simulink model "mainModel"  (R2018a)
settings: Solver=ode4  StartTime=0.0  StopTime=tsim  FixedStep=dt  RelTol=1e-3
values from neighbouring files (symbols this model uses):
  bh = 1.72    [loadParameters.m]
  Bm = 0.101    [loadParameters.m]
  Bs = 0.0602    [loadParameters.m]
  Im = 0.00136    [loadParameters.m]
  Is = 0.00129    [loadParameters.m]
  Kd = 0.1    [main.m]
  kh = 155    [loadParameters.m]
  Kp = 1.0    (= 1)    [main.m]
  L = 0.075    [loadParameters.m]
  mh = 0.1    [loadParameters.m]
  OPTION = 2    [main.m]
  wph = 87.3    [loadParameters.m]
  wzh = 98.7    [loadParameters.m]
  zph = 0.49    [loadParameters.m]
libraries: simulink_extras x1
settings Model: Creator=s118759  LastModifiedBy=s118759
settings DebuggingCC: AlgebraicLoopMsg=none

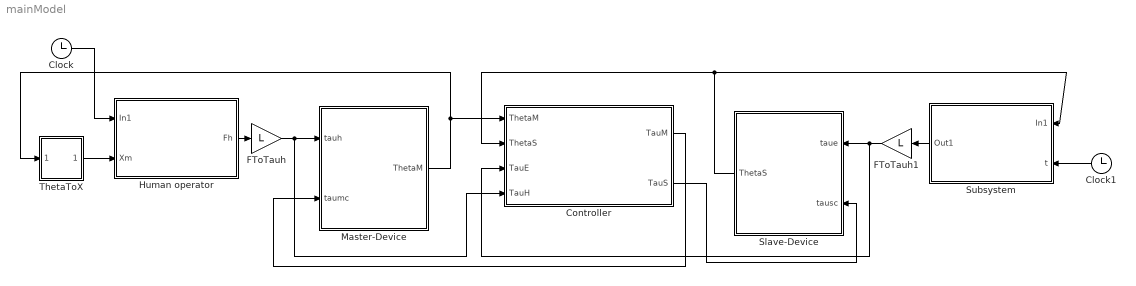
== system mainModel ==
  Clock : Clock
  Clock1 : Clock
  "Controller " : Subsystem
  FToTauh : Gain  Gain=L
  FToTauh1 : Gain  Gain=L
  "Human operator " : Subsystem
  "Master-Device " : Subsystem
  Slave-Device : Subsystem
  Subsystem : Subsystem
  "ThetaToX " : Subsystem
  wires:
  Clock/1 -> "Human operator "/1(In1)
  "Human operator "/1("Fh ") -> FToTauh/1
  FToTauh/1 -> "Master-Device "/1("tauh "), "Controller "/4("TauH ")
  "Master-Device "/1("ThetaM ") -> "Controller "/1("ThetaM "), "ThetaToX "/1(In1)
  "ThetaToX "/1(Out1) -> "Human operator "/2("Xm ")
  "Controller "/2("TauS ") -> Slave-Device/2("tausc ")
  "Controller "/1(TauM) -> "Master-Device "/2("taumc ")
  Slave-Device/1("ThetaS ") -> Subsystem/1(In1), "Controller "/2("ThetaS ")
  FToTauh1/1 -> "Controller "/3("TauE "), Slave-Device/1("taue ")
  Subsystem/1(Out1) -> FToTauh1/1
  Clock1/1 -> Subsystem/2(t)

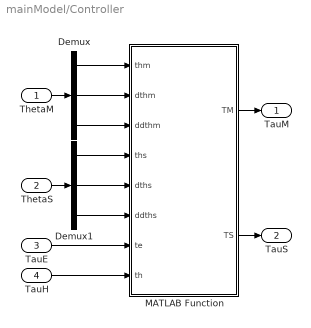
== system mainModel/Controller  ==
  "ThetaM " : Inport
  "ThetaS " : Inport  Port=2
  "TauE " : Inport  Port=3
  "TauH " : Inport  Port=4
  Demux : Demux  Outputs=3
  Demux1 : Demux  Outputs=3
  MATLAB Function : MATLAB Function  TreatAsAtomicUnit=on
  TauM : Outport
  "TauS " : Outport  Port=2
  wires:
  "ThetaM "/1 -> Demux/1
  "ThetaS "/1 -> Demux1/1
  MATLAB Function/1(TM) -> TauM/1
  MATLAB Function/2(TS) -> "TauS "/1
  Demux/3 -> MATLAB Function/3(ddthm)
  Demux/2 -> MATLAB Function/2(dthm)
  Demux/1 -> MATLAB Function/1(thm)
  Demux1/1 -> MATLAB Function/4(ths)
  Demux1/2 -> MATLAB Function/5(dths)
  Demux1/3 -> MATLAB Function/6(ddths)
  "TauH "/1 -> MATLAB Function/8(th)
  "TauE "/1 -> MATLAB Function/7(te)

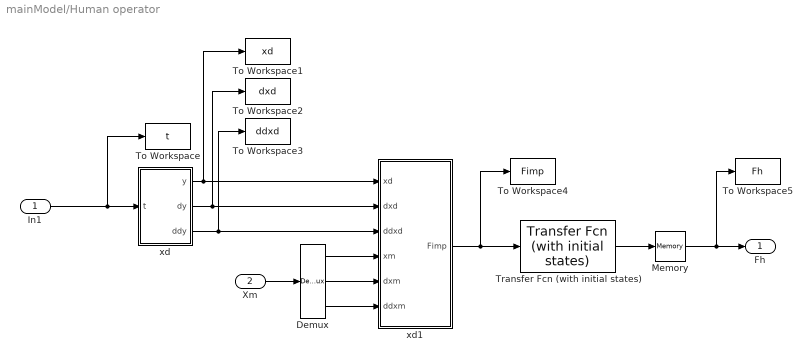
== system mainModel/Human operator  ==
  In1 : Inport
  "Xm " : Inport  Port=2
  Demux : Demux  Outputs=3
  Memory : Memory
  To Workspace : ToWorkspace  VariableName=t  SampleTime=-1
  To Workspace1 : ToWorkspace  VariableName=xd  SampleTime=-1
  To Workspace2 : ToWorkspace  VariableName=dxd  SampleTime=-1
  To Workspace3 : ToWorkspace  VariableName=ddxd  SampleTime=-1
  To Workspace4 : ToWorkspace  VariableName=Fimp  SampleTime=-1
  To Workspace5 : ToWorkspace  VariableName=Fh  SampleTime=-1
  Transfer Fcn (with initial states) : simulink_extras/Additional Linear/Transfer Fcn (with initial states)  N=[2*zph*wph, wph^2]  D=[(wph^2/wzh), wph^2]  X0=0
  xd : MATLAB Function  TreatAsAtomicUnit=on
  xd1 : MATLAB Function  TreatAsAtomicUnit=on
  "Fh " : Outport
  wires:
  In1/1 -> xd/1(t), To Workspace/1
  xd/1(y) -> To Workspace1/1, xd1/1(xd)
  xd/3(ddy) -> xd1/3(ddxd), To Workspace3/1
  xd/2(dy) -> To Workspace2/1, xd1/2(dxd)
  Demux/3 -> xd1/6(ddxm)
  Demux/2 -> xd1/5(dxm)
  Demux/1 -> xd1/4(xm)
  "Xm "/1 -> Demux/1
  xd1/1(Fimp) -> Transfer Fcn (with initial states)/1, To Workspace4/1
  Transfer Fcn (with initial states)/1 -> Memory/1
  Memory/1 -> To Workspace5/1, "Fh "/1

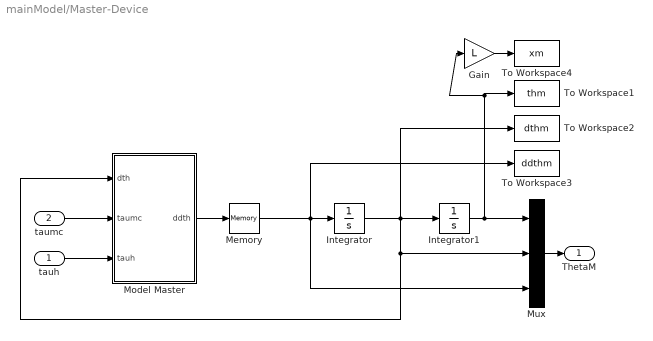
== system mainModel/Master-Device  ==
  "tauh " : Inport
  "taumc " : Inport  Port=2
  Gain : Gain  Gain=L
  Integrator : Integrator
  Integrator1 : Integrator
  Memory : Memory
  "Model Master " : MATLAB Function  TreatAsAtomicUnit=on
  Mux : Mux  Inputs=3
  To Workspace1 : ToWorkspace  VariableName=thm  SampleTime=-1
  To Workspace2 : ToWorkspace  VariableName=dthm  SampleTime=-1
  To Workspace3 : ToWorkspace  VariableName=ddthm  SampleTime=-1
  To Workspace4 : ToWorkspace  VariableName=xm  SampleTime=-1
  "ThetaM " : Outport
  wires:
  "tauh "/1 -> "Model Master "/3(tauh)
  "taumc "/1 -> "Model Master "/2(taumc)
  Integrator/1 -> To Workspace2/1, Mux/2, "Model Master "/1(dth), Integrator1/1
  Mux/1 -> "ThetaM "/1
  Integrator1/1 -> Gain/1, To Workspace1/1, Mux/1
  "Model Master "/1(ddth) -> Memory/1
  Gain/1 -> To Workspace4/1
  Memory/1 -> To Workspace3/1, Mux/3, Integrator/1

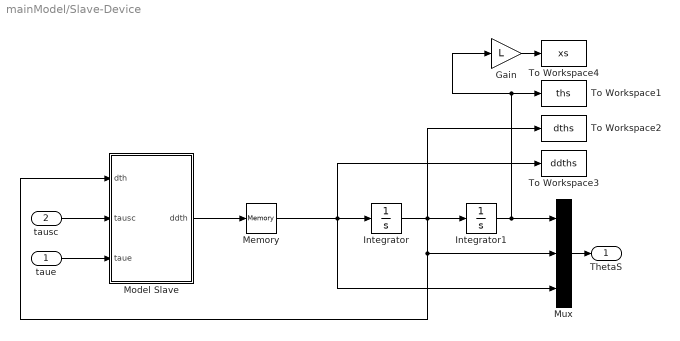
== system mainModel/Slave-Device ==
  "taue " : Inport
  "tausc " : Inport  Port=2
  Gain : Gain  Gain=L
  Integrator : Integrator
  Integrator1 : Integrator
  Memory : Memory
  "Model Slave " : MATLAB Function  TreatAsAtomicUnit=on
  Mux : Mux  Inputs=3
  To Workspace1 : ToWorkspace  VariableName=ths  SampleTime=-1
  To Workspace2 : ToWorkspace  VariableName=dths  SampleTime=-1
  To Workspace3 : ToWorkspace  VariableName=ddths  SampleTime=-1
  To Workspace4 : ToWorkspace  VariableName=xs  SampleTime=-1
  "ThetaS " : Outport
  wires:
  "taue "/1 -> "Model Slave "/3(taue)
  "tausc "/1 -> "Model Slave "/2(tausc)
  Integrator/1 -> To Workspace2/1, Mux/2, "Model Slave "/1(dth), Integrator1/1
  Mux/1 -> "ThetaS "/1
  Integrator1/1 -> Gain/1, To Workspace1/1, Mux/1
  "Model Slave "/1(ddth) -> Memory/1
  Gain/1 -> To Workspace4/1
  Memory/1 -> To Workspace3/1, Mux/3, Integrator/1

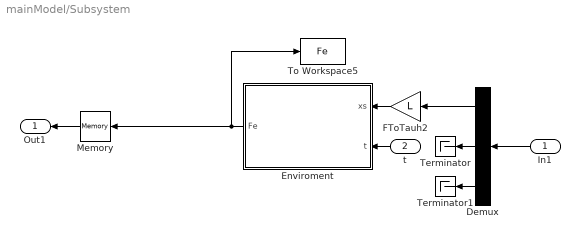
== system mainModel/Subsystem ==
  In1 : Inport
  t : Inport  Port=2
  Demux : Demux  Outputs=3
  "Enviroment " : MATLAB Function  TreatAsAtomicUnit=on
  FToTauh2 : Gain  Gain=L
  Memory : Memory
  Terminator : Terminator
  Terminator1 : Terminator
  To Workspace5 : ToWorkspace  VariableName=Fe  SampleTime=-1
  Out1 : Outport
  wires:
  FToTauh2/1 -> "Enviroment "/1(xs)
  "Enviroment "/1(Fe) -> To Workspace5/1, Memory/1
  Demux/1 -> FToTauh2/1
  In1/1 -> Demux/1
  Demux/2 -> Terminator/1
  Demux/3 -> Terminator1/1
  Memory/1 -> Out1/1
  t/1 -> "Enviroment "/2(t)

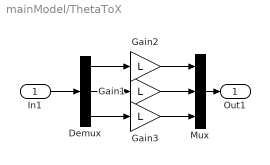
== system mainModel/ThetaToX  ==
  In1 : Inport
  Demux : Demux  Outputs=3
  Gain1 : Gain  Gain=L
  Gain2 : Gain  Gain=L
  Gain3 : Gain  Gain=L
  Mux : Mux  Inputs=3
  Out1 : Outport
  wires:
  In1/1 -> Demux/1
  Mux/1 -> Out1/1
  Demux/1 -> Gain2/1
  Gain1/1 -> Mux/2
  Demux/2 -> Gain1/1
  Gain2/1 -> Mux/1
  Demux/3 -> Gain3/1
  Gain3/1 -> Mux/3

== matlab function mainModel/Human operator /xd1 ==
  data: xd input; dxd input; ddxd input; Fimp output; xm input; dxm input; ddxm input; mh parameter; bh parameter; kh parameter
function Fimp = fcn(xd,dxd,ddxd,xm,dxm,ddxm,mh,bh,kh)
Fimp = kh*(xd-xm) + bh*(dxd-dxm) + mh*(ddxd - ddxm);
end

== matlab function mainModel/Human operator /xd ==
  data: t input; y output; dy output; ddy output
function [y,dy,ddy] = fcn(t)
y   = -0.015*sin(0.75*pi*t) -0.03*sin(0.25*pi*t);
dy  = - (3*pi*cos((pi*t)/4))/400 - (9*pi*cos((3*pi*t)/4))/800;
ddy = (3*pi^2*sin((pi*t)/4))/1600 + (27*pi^2*sin((3*pi*t)/4))/3200;

== matlab function mainModel/Master-Device /Model Master  ==
  data: dth input; taumc input; tauh input; ddth output; Im parameter; Bm parameter
function ddth = fcn(dth,taumc,tauh,Im,Bm)

ddth = (1/Im)*(tauh + taumc - Bm*dth);

end

== matlab function mainModel/Slave-Device/Model Slave  ==
  data: dth input; tausc input; taue input; ddth output; Is parameter; Bs parameter
function ddth = fcn(dth,tausc,taue,Is,Bs)
ddth = (1/Is)*(-taue + tausc - Bs*dth);
end

== matlab function mainModel/Subsystem/Enviroment  ==
  data: xs input; Fe output; ke parameter; t input
function Fe = fcn(xs,ke,t)
if(xs <= 0), Fe = 0;
else, Fe = ke*xs;
end

== matlab function mainModel/Controller /MATLAB Function ==
  data: thm input; TM output; dthm input; ddthm input; ths input; dths input; ddths input; te input; th input; TS output; Kd parameter; Kp parameter; OPTION parameter
function [TM,TS] = fcn(thm,dthm,ddthm,ths,dths,ddths,te,th,Kd,Kp,OPTION)

if(OPTION == 1)
    TM = Kp*(ths-thm) + Kd*(dths-dthm);
    TS = Kp*(thm-ths) + Kd*(dthm-dths);
elseif(OPTION == 2)
    TM = -te;
    TS = Kp*(thm-ths) + Kd*(dthm-dths);
elseif(OPTION == 3)
    TM = -te;
    TS = th;
else
    TM = 0;
    TS = 0;
end

end
